simulink model "V511_L5_TDI"  (R2023b)
settings: Solver=VariableStepAuto  StartTime=0.0  StopTime=200  MaxStep=0.01  RelTol=1e-3
values from neighbouring files (symbols this model uses):
  acs = ap+K*bp    [pz5.m]
  ap = Wp.Denominator{1}    [pz5.m]
  bp = Wp.Numerator{1}    [pz5.m]
  K = 20    [DMikh.m]    (also in pz5.m = 35)
  K1 = 0.5    [pz5.m]
  K2 = 0.1    [pz5.m]
  mcs = mp+K*np    [DMikh.m]    (also in pz5.m)
  mp = Wpzoh.Denominator{1}    [pz5.m]
  np = Wpzoh.Numerator{1}    [pz5.m]
  q = 0.2    [pz5.m]
  T1 = 4    [pz5.m]
  T2 = 5    [pz5.m]
  T3 = 1    [pz5.m]
  Ts = 0.1* (T1 + T2 + T3)    (= 1)    [pz5.m]
  Un = 80    [pz5.m]
settings Model: Creator=td  LastModifiedBy=killer
settings SolverCC: AlgebraicLoopSolver=TrustRegion
settings DataIOCC: ReturnWorkspaceOutputs=off
settings DebuggingCC: UnconnectedInputMsg=warning  UnconnectedOutputMsg=warning  UnconnectedLineMsg=warning  ArithmeticOperatorsInVariantConditions=warning
settings ModelReferenceCC: EnableRefExpFcnMdlSchedulingChecks=on
settings SFSimCC: CustomCodeUndefinedFunction=UseInterfaceOnly

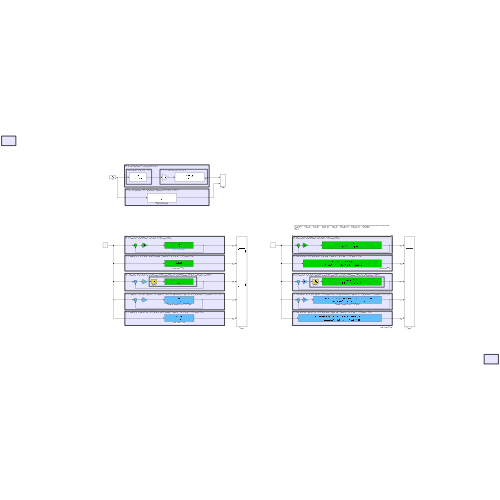
[thumbnail: Simulink's stored preview of the top-level diagram]
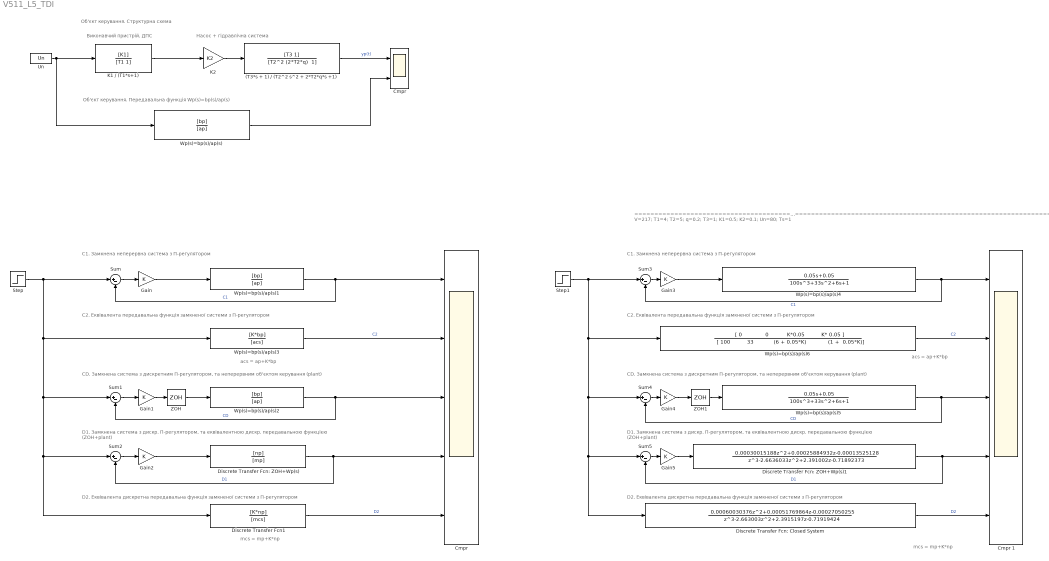
== system V511_L5_TDI ==
  note: =======================================================================================================
      | V=217; T1=4; T2=5; q=0.2; T3=1; K1=0.5; K2=0.1; Un=80;
      | Ts=1
  note: acs = ap+K*bp
  note: С1. Замкнена неперервна система з П-регулятором
  note: mcs = mp+K*np
  note: Насос + гідравлічна система
  note: Об'єкт керування. Структурна схема
  note: Виконавчий пристрій, ДПС
  note: Об'єкт керування. Передавальна функція Wp(s)=bp(s)/ap(s)
  note: С2. Еквівалента передавальна функція замкненої системи з П-регулятором
  note: СD. Замкнена система з дискретним П-регулятором, та неперервним об'єктом керування (plant)
  note: D1. Замкнена система з дискр. П-регулятором, та еквівалентною дискр. передавальною функцією (ZOH+plant)
  note: D2. Еквівалента дискретна передавальна функція замкненої системи з П-регулятором
  note: С1. Замкнена неперервна система з П-регулятором
  note: СD. Замкнена система з дискретним П-регулятором, та неперервним об'єктом керування (plant)
  note: С2. Еквівалента передавальна функція замкненої системи з П-регулятором
  note: mcs = mp+K*np
  note: D1. Замкнена система з дискр. П-регулятором, та еквівалентною дискр. передавальною функцією (ZOH+plant)
  note: D2. Еквівалента дискретна передавальна функція замкненої системи з П-регулятором
  note: acs = ap+K*bp
  " Discrete Transfer Fcn: Closed System" : DiscreteTransferFcn  Numerator="[ 0  0.00060030376  0.00051769864 -0.00027050255 ]"  Denominator="[ 1      -2.663003      2.3915197    -0.71919424 ]"  SampleTime=Ts
  " Discrete Transfer Fcn: ZOH+Wp(s)" : DiscreteTransferFcn  Numerator=[np]  Denominator=[mp]  SampleTime=Ts
  " Discrete Transfer Fcn: ZOH+Wp(s)1" : DiscreteTransferFcn  Numerator="[ 0  0.00030015188  0.00025884932 -0.00013525128 ]"  Denominator="[ 1     -2.6636033       2.391002    -0.71892373 ]"  SampleTime=Ts
  (T3*s + 1) / (T2^2 s^2 + 2*T2*q*s +1) : TransferFcn  Numerator=[T3 1]  Denominator="[T2^2 (2*T2*q)  1]"
  Cmpr : Scope  NumInputPorts=2
  "Cmpr " : Scope  NumInputPorts=5
  Cmpr 1 : Scope  NumInputPorts=5
  Discrete Transfer Fcn1 : DiscreteTransferFcn  Numerator=[K*np]  Denominator=[mcs]  SampleTime=Ts
  Gain{,1..5} (6 alike) : Gain  Gain=K
  K1 / (T1*s+1) : TransferFcn  Numerator=[K1]  Denominator=[T1 1]
  K2 : Gain  Gain=K2
  Step : Step  SampleTime=0
  Step1 : Step  SampleTime=0
  Sum{,1..5} (6 alike) : Sum  Inputs=|+-
  Un : Constant  Value=Un
  Wp(s)=bp(s)/ap(s) : TransferFcn  Numerator=[bp]  Denominator=[ap]
  Wp(s)=bp(s)/ap(s)1 : TransferFcn  Numerator=[bp]  Denominator=[ap]
  Wp(s)=bp(s)/ap(s)2 : TransferFcn  Numerator=[bp]  Denominator=[ap]
  Wp(s)=bp(s)/ap(s)3 : TransferFcn  Numerator=[K*bp]  Denominator=[acs]
  Wp(s)=bp(s)/ap(s)4 : TransferFcn  Numerator="[ 0              0           0.05           0.05 ]"  Denominator="[ 100             33              6              1 ]"
  Wp(s)=bp(s)/ap(s)5 : TransferFcn  Numerator=[ 0 0 0.05 0.05]  Denominator="[ 100             33           6           1 ]"
  Wp(s)=bp(s)/ap(s)6 : TransferFcn  Numerator="[ 0              0           K*0.05          K* 0.05 ]"  Denominator="[ 100          33            (6 + 0.05*K)             (1 +  0.05*K)]"
  ZOH : ZeroOrderHold  SampleTime=Ts
  ZOH1 : ZeroOrderHold  SampleTime=Ts
  wires:
  Un/1 -> Wp(s)=bp(s)/ap(s)/1, K1 / (T1*s+1)/1
  K2/1 -> (T3*s + 1) / (T2^2 s^2 + 2*T2*q*s +1)/1
  (T3*s + 1) / (T2^2 s^2 + 2*T2*q*s +1)/1 -> Cmpr/1  "yp(t)"
  K1 / (T1*s+1)/1 -> K2/1
  Wp(s)=bp(s)/ap(s)/1 -> Cmpr/2
  Wp(s)=bp(s)/ap(s)1/1 -> Sum/2, "Cmpr "/1  "C1"
  Wp(s)=bp(s)/ap(s)2/1 -> Sum1/2, "Cmpr "/3  "CD"
  Step/1 -> Sum/1, Sum1/1, Sum2/1, Discrete Transfer Fcn1/1, Wp(s)=bp(s)/ap(s)3/1
  ZOH/1 -> Wp(s)=bp(s)/ap(s)2/1
  Sum/1 -> Gain/1
  Gain/1 -> Wp(s)=bp(s)/ap(s)1/1
  Sum1/1 -> Gain1/1
  Gain1/1 -> ZOH/1
  Gain2/1 -> " Discrete Transfer Fcn: ZOH+Wp(s)"/1
  Sum2/1 -> Gain2/1
  " Discrete Transfer Fcn: ZOH+Wp(s)"/1 -> Sum2/2, "Cmpr "/4  "D1"
  Wp(s)=bp(s)/ap(s)3/1 -> "Cmpr "/2  "C2"
  Discrete Transfer Fcn1/1 -> "Cmpr "/5  "D2"
  Wp(s)=bp(s)/ap(s)5/1 -> Cmpr 1/3, Sum4/2  "CD"
  " Discrete Transfer Fcn: ZOH+Wp(s)1"/1 -> Sum5/2, Cmpr 1/4  "D1"
  Gain4/1 -> ZOH1/1
  Sum3/1 -> Gain3/1
  Gain3/1 -> Wp(s)=bp(s)/ap(s)4/1
  Wp(s)=bp(s)/ap(s)6/1 -> Cmpr 1/2  "C2"
  Sum4/1 -> Gain4/1
  Gain5/1 -> " Discrete Transfer Fcn: ZOH+Wp(s)1"/1
  Wp(s)=bp(s)/ap(s)4/1 -> Sum3/2, Cmpr 1/1  "C1"
  Step1/1 -> " Discrete Transfer Fcn: Closed System"/1, Sum5/1, Sum4/1, Wp(s)=bp(s)/ap(s)6/1, Sum3/1
  Sum5/1 -> Gain5/1
  ZOH1/1 -> Wp(s)=bp(s)/ap(s)5/1
  " Discrete Transfer Fcn: Closed System"/1 -> Cmpr 1/5  "D2"
